simulink model "LogicalOperator"  (R2015b)
settings: Solver=VariableStepAuto  StartTime=0.0  StopTime=10.0  RelTol=1e-3
settings Model: Creator=LUBO  LastModifiedBy=LUBO

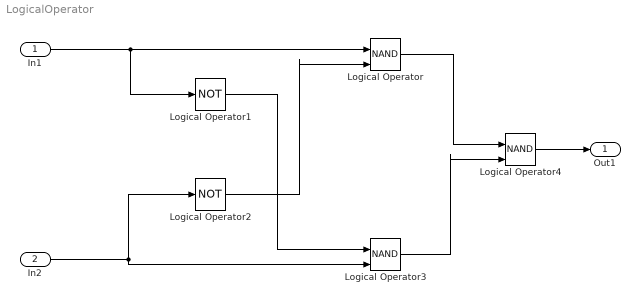
== system LogicalOperator ==
  In1 : Inport
  In2 : Inport  Port=2
  Logical Operator : Logic  Operator=NAND  IconShape=distinctive  AllPortsSameDT=off  OutDataTypeStr=boolean
  Logical Operator1 : Logic  Operator=NOT  IconShape=distinctive  AllPortsSameDT=off  OutDataTypeStr=boolean
  Logical Operator2 : Logic  Operator=NOT  IconShape=distinctive  AllPortsSameDT=off  OutDataTypeStr=boolean
  Logical Operator3 : Logic  Operator=NAND  IconShape=distinctive  AllPortsSameDT=off  OutDataTypeStr=boolean
  Logical Operator4 : Logic  Operator=NAND  IconShape=distinctive  AllPortsSameDT=off  OutDataTypeStr=boolean
  Out1 : Outport
  wires:
  In1/1 -> Logical Operator/1, Logical Operator1/1
  In2/1 -> Logical Operator3/2, Logical Operator2/1
  Logical Operator2/1 -> Logical Operator/2
  Logical Operator1/1 -> Logical Operator3/1
  Logical Operator/1 -> Logical Operator4/1
  Logical Operator3/1 -> Logical Operator4/2
  Logical Operator4/1 -> Out1/1
